simulink model "GreenCraneSimulator_SomplifiedHydMechModel"  (R2021b)
settings: Solver=ode23  StartTime=0.0  StopTime=25  FixedStep=0.0001  RelTol=1e-3
undefined symbols (not defined in the file): DiscIntNeverNeededParam, tCycle, X, Y, Z
libraries: sm_lib x25, nesl_utility x4, simulink x1
(part 1 of 2)
settings Model: Creator=hagen  LastModifiedBy=danielh

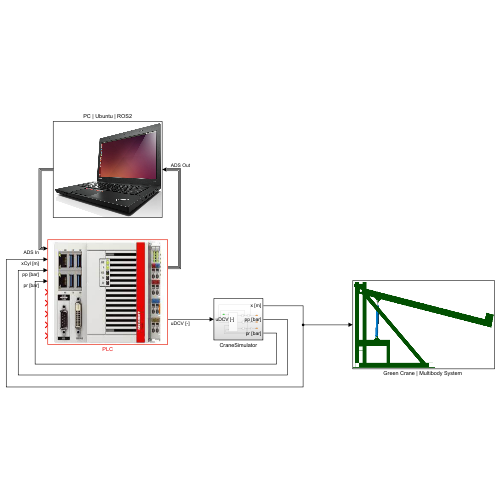
[thumbnail: Simulink's stored preview of the top-level diagram]
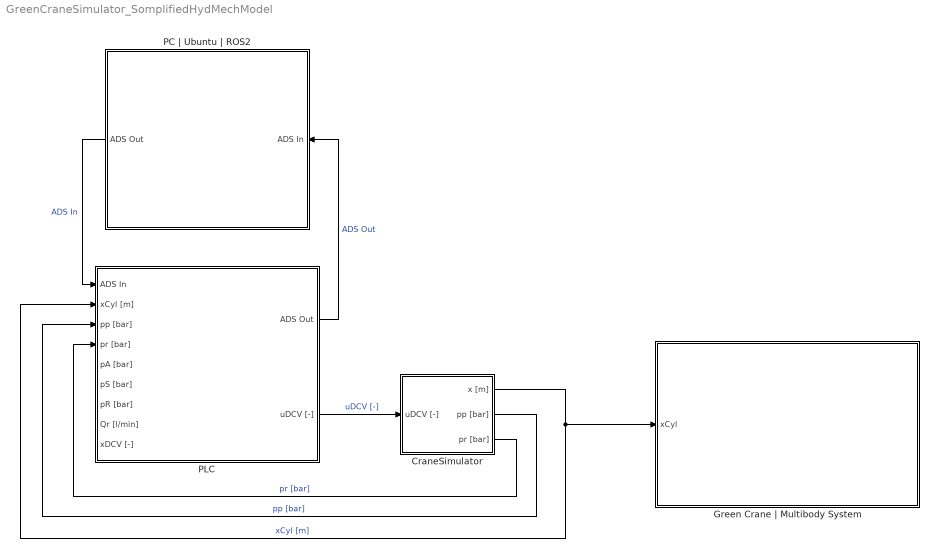
== system GreenCraneSimulator_SomplifiedHydMechModel ==
  CraneSimulator : Subsystem
  "Green Crane | Multibody System " : Subsystem
      mask Display: image('..\MAS418_SimulinkModel\Figures\GreenCrane.png'); % Use "Edit Image" on toolstrip to change.
  PC | Ubuntu | ROS2 : Subsystem
      mask Display: image('..\MAS418_SimulinkModel\Figures\PC.png'); % Use "Edit Image" on toolstrip to change.
  PLC : Subsystem
      mask Display: image('..\MAS418_SimulinkModel\Figures\PLC.jpg'); % Use "Edit Image" on toolstrip to change.
  wires:
  PC | Ubuntu | ROS2/1(ADS Out) -> PLC/1(ADS In)  "ADS In"
  CraneSimulator/2(pp [bar]) -> PLC/3(pp [bar])  "pp [bar]"
  CraneSimulator/3(pr [bar]) -> PLC/4(pr [bar])  "pr [bar]"
  PLC/1(ADS Out) -> PC | Ubuntu | ROS2/1(ADS In)  "ADS Out"
  PLC/2(uDCV [-]) -> CraneSimulator/1(uDCV [-])  "uDCV [-]"
  CraneSimulator/1(x [m]) -> PLC/2(xCyl [m]), "Green Crane | Multibody System "/1(xCyl)  "xCyl [m]"

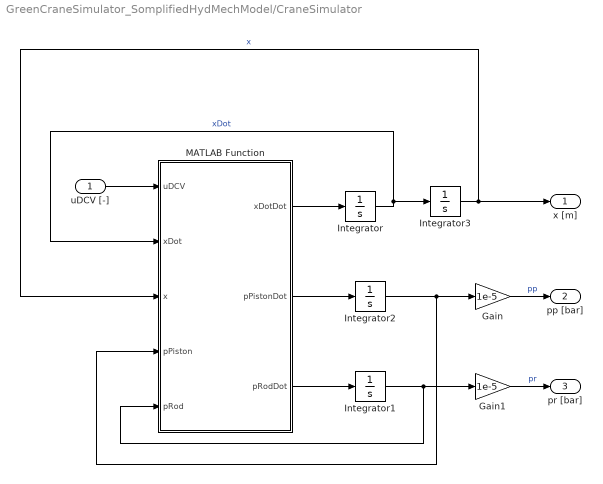
== system GreenCraneSimulator_SomplifiedHydMechModel/CraneSimulator ==
  uDCV [-] : Inport
  Gain : Gain  Gain=1e-5
  Gain1 : Gain  Gain=1e-5
  Integrator : Integrator  LimitOutput=on  UpperSaturationLimit=0.12  LowerSaturationLimit=-0.12
  Integrator1 : Integrator  InitialCondition=4.683e5  LimitOutput=on  UpperSaturationLimit=180e5  LowerSaturationLimit=1.1e5
  Integrator2 : Integrator  InitialCondition=43.77e5  LimitOutput=on  UpperSaturationLimit=180e5  LowerSaturationLimit=1.1e5
  Integrator3 : Integrator  LimitOutput=on  UpperSaturationLimit=0.5  LowerSaturationLimit=0
  MATLAB Function : MATLAB Function  TreatAsAtomicUnit=on
  x [m] : Outport
  pp [bar] : Outport  Port=2
  pr [bar] : Outport  Port=3
  wires:
  uDCV [-]/1 -> MATLAB Function/1(uDCV)
  MATLAB Function/2(pPistonDot) -> Integrator2/1
  Integrator3/1 -> x [m]/1, MATLAB Function/3(x)  "x"
  Integrator2/1 -> Gain/1, MATLAB Function/4(pPiston)
  Integrator/1 -> Integrator3/1, MATLAB Function/2(xDot)  "xDot"
  Integrator1/1 -> Gain1/1, MATLAB Function/5(pRod)
  Gain/1 -> pp [bar]/1  "pp"
  MATLAB Function/3(pRodDot) -> Integrator1/1
  MATLAB Function/1(xDotDot) -> Integrator/1
  Gain1/1 -> pr [bar]/1  "pr"

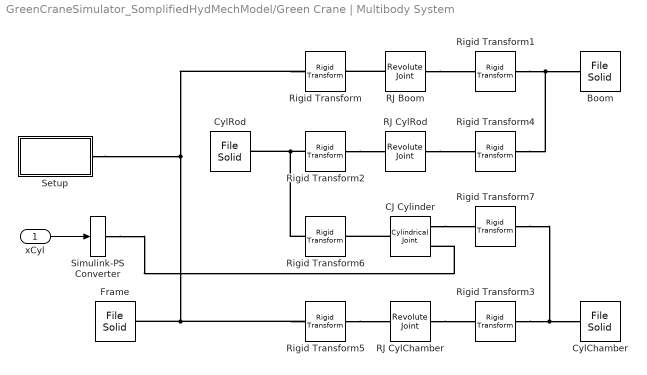
== system GreenCraneSimulator_SomplifiedHydMechModel/Green Crane | Multibody System  ==
  xCyl : Inport
  Boom : sm_lib/Body Elements/File Solid  ExtGeomFileName=..\MAS418_SimulinkModel\CAD\Boom.STL  UnitType=Custom  ExtGeomFileUnits=mm  StepReaderType=HEX  ExportConvexHullGeometry=off  InertiaType=CalculateFromGeometry  Mass=1  MassUnits=kg  CenterOfMass=[0 0 0]  CenterOfMassUnits=m  MomentsOfInertia=[1 1 1]  MomentsOfInertiaUnits=kg*m^2  ProductsOfInertia=[0 0 0]  ProductsOfInertiaUnits=kg*m^2  BasedOnType=Density  Density=1000  DensityUnits=kg/m^3  DoExposeReferenceFrame=off  SerializedFrames=<Frames><Frame><Id>Frame1</Id><Value><Name>F1</Name><Origin><Source>CenterOfMassFrame</Source><FeatureName></FeatureName></Origin><PrimaryAxis><DefinedDirection>+Y</DefinedDirection><Source>ReferenceFrame</Source><SourceDirection>-Z</SourceDirection><FeatureName></FeatureName></PrimaryAxis><SecondaryAxis><DefinedDirection>+X</DefinedDirection><Source>ReferenceFrame</Source><SourceDirection>+X</SourceDirection><FeatureName></FeatureName></SecondaryAxis></Value></Frame></Frames>  GraphicType=FromGeometry  MarkerShape=Sphere  MarkerSize=10  GraphicVisPropType=SimpleVisualProperties  GraphicDiffuseColor=[0.0 0.4 0.0]  GraphicSpecularColor=[0.5 0.5 0.5 1.0]  GraphicAmbientColor=[0.15 0.15 0.15 1.0]  GraphicEmissiveColor=[0.0 0.0 0.0 1.0]  GraphicShininess=75  GraphicOpacity=1.0
  CJ Cylinder : sm_lib/Joints/Cylindrical Joint  JointMode=Normal  SenseConstraintForce=off  SenseConstraintForceX=off  SenseConstraintForceY=off  SenseConstraintForceZ=off  SenseConstraintTorque=off  SenseConstraintTorqueX=off  SenseConstraintTorqueY=off  SenseConstraintTorqueZ=off  SenseTotalForce=off  SenseTotalForceX=off  SenseTotalForceY=off  SenseTotalForceZ=off  SenseTotalTorque=off  SenseTotalTorqueX=off  SenseTotalTorqueY=off  SenseTotalTorqueZ=off  CompositeWrenchDir=FollowerOnBase  CompositeWrenchFrame=BaseFrame  PzEquilibriumPosition=0  PzEquilibriumPositionUnits=m  PzSpringStiffness=0  PzSpringStiffnessUnits=N/m  PzDampingCoefficient=0  PzDampingCoefficientUnits=N/(m/s)  PzTorqueActuationMode=ComputedTorque  PzMotionActuationMode=InputMotion  PzSensePosition=off  PzSenseVelocity=off  PzSenseAcceleration=off  PzSenseTorqueForce=off  PzSenseLowerLimitTorqueForce=off  PzSenseUpperLimitTorqueForce=off  PzLowerLimitSpecify=off  PzLowerLimitBound=-1  PzLowerLimitBoundUnits=m  PzLowerLimitStiffness=1e6  PzLowerLimitStiffnessUnits=N/m  PzLowerLimitDamping=1e3  PzLowerLimitDampingUnits=N/(m/s)  PzLowerLimitTransitionRegionWidth=1e-4  PzLowerLimitTransitionRegionWidthUnits=m  PzUpperLimitSpecify=off  PzUpperLimitBound=1  PzUpperLimitBoundUnits=m  PzUpperLimitStiffness=1e6  PzUpperLimitStiffnessUnits=N/m  PzUpperLimitDamping=1e3  PzUpperLimitDampingUnits=N/(m/s)  PzUpperLimitTransitionRegionWidth=1e-4  PzUpperLimitTransitionRegionWidthUnits=m  PzPositionTargetSpecify=on  PzPositionTargetPriority=High  PzPositionTargetValue=0  PzPositionTargetValueUnits=m  PzVelocityTargetSpecify=off  PzVelocityTargetPriority=High  PzVelocityTargetValue=0  PzVelocityTargetValueUnits=m/s  RzEquilibriumPosition=0  RzEquilibriumPositionUnits=deg  RzSpringStiffness=0  RzSpringStiffnessUnits=N*m/deg  RzDampingCoefficient=0  RzDampingCoefficientUnits=N*m/(deg/s)  RzTorqueActuationMode=NoTorque  RzMotionActuationMode=ComputedMotion  RzSensePosition=off  RzSenseVelocity=off  RzSenseAcceleration=off  RzSenseTorqueForce=off  RzSenseLowerLimitTorqueForce=off  RzSenseUpperLimitTorqueForce=off  RzLowerLimitSpecify=off  RzLowerLimitBound=-90  RzLowerLimitBoundUnits=deg  RzLowerLimitStiffness=1e4  RzLowerLimitStiffnessUnits=N*m/deg  RzLowerLimitDamping=10  RzLowerLimitDampingUnits=N*m/(deg/s)  RzLowerLimitTransitionRegionWidth=0.1  RzLowerLimitTransitionRegionWidthUnits=deg  RzUpperLimitSpecify=off  RzUpperLimitBound=90  RzUpperLimitBoundUnits=deg  RzUpperLimitStiffness=1e4  RzUpperLimitStiffnessUnits=N*m/deg  RzUpperLimitDamping=10  RzUpperLimitDampingUnits=N*m/(deg/s)  RzUpperLimitTransitionRegionWidth=0.1  RzUpperLimitTransitionRegionWidthUnits=deg  RzPositionTargetSpecify=off  RzPositionTargetPriority=High  RzPositionTargetValue=0  RzPositionTargetValueUnits=deg  RzVelocityTargetSpecify=off  RzVelocityTargetPriority=High  RzVelocityTargetValue=0  RzVelocityTargetValueUnits=deg/s
  CylChamber : sm_lib/Body Elements/File Solid  ExtGeomFileName=..\MAS418_SimulinkModel\CAD\cyl_chamber.STL  UnitType=Custom  ExtGeomFileUnits=mm  StepReaderType=HEX  ExportConvexHullGeometry=off  InertiaType=CalculateFromGeometry  Mass=1  MassUnits=kg  CenterOfMass=[0 0 0]  CenterOfMassUnits=m  MomentsOfInertia=[1 1 1]  MomentsOfInertiaUnits=kg*m^2  ProductsOfInertia=[0 0 0]  ProductsOfInertiaUnits=kg*m^2  BasedOnType=Density  Density=1000  DensityUnits=kg/m^3  DoExposeReferenceFrame=off  SerializedFrames=<Frames><Frame><Id>Frame1</Id><Value><Name>F1</Name><Origin><Source>CenterOfMassFrame</Source><FeatureName></FeatureName></Origin><PrimaryAxis><DefinedDirection>+Y</DefinedDirection><Source>ReferenceFrame</Source><SourceDirection>-Z</SourceDirection><FeatureName></FeatureName></PrimaryAxis><SecondaryAxis><DefinedDirection>+X</DefinedDirection><Source>ReferenceFrame</Source><SourceDirection>+X</SourceDirection><FeatureName></FeatureName></SecondaryAxis></Value></Frame></Frames>  GraphicType=FromGeometry  MarkerShape=Sphere  MarkerSize=10  GraphicVisPropType=SimpleVisualProperties  GraphicDiffuseColor=[0.0 0.6 1.0]  GraphicSpecularColor=[0.5 0.5 0.5 1.0]  GraphicAmbientColor=[0.15 0.15 0.15 1.0]  GraphicEmissiveColor=[0.0 0.0 0.0 1.0]  GraphicShininess=75  GraphicOpacity=1.0
  CylRod : sm_lib/Body Elements/File Solid  ExtGeomFileName=..\MAS418_SimulinkModel\CAD\cyl_rod.STL  UnitType=Custom  ExtGeomFileUnits=mm  StepReaderType=HEX  ExportConvexHullGeometry=off  InertiaType=CalculateFromGeometry  Mass=1  MassUnits=kg  CenterOfMass=[0 0 0]  CenterOfMassUnits=m  MomentsOfInertia=[1 1 1]  MomentsOfInertiaUnits=kg*m^2  ProductsOfInertia=[0 0 0]  ProductsOfInertiaUnits=kg*m^2  BasedOnType=Density  Density=1000  DensityUnits=kg/m^3  DoExposeReferenceFrame=off  SerializedFrames=<Frames><Frame><Id>Frame1</Id><Value><Name>F1</Name><Origin><Source>CenterOfMassFrame</Source><FeatureName></FeatureName></Origin><PrimaryAxis><DefinedDirection>+Y</DefinedDirection><Source>ReferenceFrame</Source><SourceDirection>-Z</SourceDirection><FeatureName></FeatureName></PrimaryAxis><SecondaryAxis><DefinedDirection>+X</DefinedDirection><Source>ReferenceFrame</Source><SourceDirection>+X</SourceDirection><FeatureName></FeatureName></SecondaryAxis></Value></Frame></Frames>  GraphicType=FromGeometry  MarkerShape=Sphere  MarkerSize=10  GraphicVisPropType=SimpleVisualProperties  GraphicDiffuseColor=[0.8 0.8 0.8]  GraphicSpecularColor=[0.5 0.5 0.5 1.0]  GraphicAmbientColor=[0.15 0.15 0.15 1.0]  GraphicEmissiveColor=[0.0 0.0 0.0 1.0]  GraphicShininess=75  GraphicOpacity=1.0
  Frame : sm_lib/Body Elements/File Solid  ExtGeomFileName=..\MAS418_SimulinkModel\CAD\Frame.STL  UnitType=Custom  ExtGeomFileUnits=mm  StepReaderType=HEX  ExportConvexHullGeometry=off  InertiaType=CalculateFromGeometry  Mass=1  MassUnits=kg  CenterOfMass=[0 0 0]  CenterOfMassUnits=m  MomentsOfInertia=[1 1 1]  MomentsOfInertiaUnits=kg*m^2  ProductsOfInertia=[0 0 0]  ProductsOfInertiaUnits=kg*m^2  BasedOnType=Density  Density=1000  DensityUnits=kg/m^3  DoExposeReferenceFrame=off  SerializedFrames=<Frames><Frame><Id>Frame1</Id><Value><Name>F1</Name><Origin><Source>CenterOfMassFrame</Source><FeatureName></FeatureName></Origin><PrimaryAxis><DefinedDirection>-Y</DefinedDirection><Source>ReferenceFrame</Source><SourceDirection>+Z</SourceDirection><FeatureName></FeatureName></PrimaryAxis><SecondaryAxis><DefinedDirection>+X</DefinedDirection><Source>ReferenceFrame</Source><SourceDirection>+X</SourceDirection><FeatureName></FeatureName></SecondaryAxis></Value></Frame></Frames>  GraphicType=FromGeometry  MarkerShape=Sphere  MarkerSize=10  GraphicVisPropType=SimpleVisualProperties  GraphicDiffuseColor=[0.0 0.4 0.0]  GraphicSpecularColor=[0.5 0.5 0.5 1.0]  GraphicAmbientColor=[0.15 0.15 0.15 1.0]  GraphicEmissiveColor=[0.0 0.0 0.0 1.0]  GraphicShininess=75  GraphicOpacity=1.0
  RJ Boom : sm_lib/Joints/Revolute Joint  JointMode=Normal  SenseConstraintForce=off  SenseConstraintForceX=off  SenseConstraintForceY=off  SenseConstraintForceZ=off  SenseConstraintTorque=off  SenseConstraintTorqueX=off  SenseConstraintTorqueY=off  SenseConstraintTorqueZ=off  SenseTotalForce=off  SenseTotalForceX=off  SenseTotalForceY=off  SenseTotalForceZ=off  SenseTotalTorque=off  SenseTotalTorqueX=off  SenseTotalTorqueY=off  SenseTotalTorqueZ=off  CompositeWrenchDir=FollowerOnBase  CompositeWrenchFrame=BaseFrame  EquilibriumPosition=0  EquilibriumPositionUnits=deg  SpringStiffness=0  SpringStiffnessUnits=N*m/deg  DampingCoefficient=0  DampingCoefficientUnits=N*m/(deg/s)  TorqueActuationMode=NoTorque  MotionActuationMode=ComputedMotion  SensePosition=off  SenseVelocity=off  SenseAcceleration=off  SenseTorqueForce=off  SenseLowerLimitTorqueForce=off  SenseUpperLimitTorqueForce=off  LowerLimitSpecify=off  LowerLimitBound=-90  LowerLimitBoundUnits=deg  LowerLimitStiffness=1e4  LowerLimitStiffnessUnits=N*m/deg  LowerLimitDamping=10  LowerLimitDampingUnits=N*m/(deg/s)  LowerLimitTransitionRegionWidth=0.1  LowerLimitTransitionRegionWidthUnits=deg  UpperLimitSpecify=off  UpperLimitBound=90  UpperLimitBoundUnits=deg  UpperLimitStiffness=1e4  UpperLimitStiffnessUnits=N*m/deg  UpperLimitDamping=10  UpperLimitDampingUnits=N*m/(deg/s)  UpperLimitTransitionRegionWidth=0.1  UpperLimitTransitionRegionWidthUnits=deg  PositionTargetSpecify=off  PositionTargetPriority=High  PositionTargetValue=0  PositionTargetValueUnits=deg  VelocityTargetSpecify=off  VelocityTargetPriority=High  VelocityTargetValue=0  VelocityTargetValueUnits=deg/s
  RJ CylChamber : sm_lib/Joints/Revolute Joint  JointMode=Normal  SenseConstraintForce=off  SenseConstraintForceX=off  SenseConstraintForceY=off  SenseConstraintForceZ=off  SenseConstraintTorque=off  SenseConstraintTorqueX=off  SenseConstraintTorqueY=off  SenseConstraintTorqueZ=off  SenseTotalForce=off  SenseTotalForceX=off  SenseTotalForceY=off  SenseTotalForceZ=off  SenseTotalTorque=off  SenseTotalTorqueX=off  SenseTotalTorqueY=off  SenseTotalTorqueZ=off  CompositeWrenchDir=FollowerOnBase  CompositeWrenchFrame=BaseFrame  EquilibriumPosition=0  EquilibriumPositionUnits=deg  SpringStiffness=0  SpringStiffnessUnits=N*m/deg  DampingCoefficient=0  DampingCoefficientUnits=N*m/(deg/s)  TorqueActuationMode=NoTorque  MotionActuationMode=ComputedMotion  SensePosition=off  SenseVelocity=off  SenseAcceleration=off  SenseTorqueForce=off  SenseLowerLimitTorqueForce=off  SenseUpperLimitTorqueForce=off  LowerLimitSpecify=off  LowerLimitBound=-90  LowerLimitBoundUnits=deg  LowerLimitStiffness=1e4  LowerLimitStiffnessUnits=N*m/deg  LowerLimitDamping=10  LowerLimitDampingUnits=N*m/(deg/s)  LowerLimitTransitionRegionWidth=0.1  LowerLimitTransitionRegionWidthUnits=deg  UpperLimitSpecify=off  UpperLimitBound=90  UpperLimitBoundUnits=deg  UpperLimitStiffness=1e4  UpperLimitStiffnessUnits=N*m/deg  UpperLimitDamping=10  UpperLimitDampingUnits=N*m/(deg/s)  UpperLimitTransitionRegionWidth=0.1  UpperLimitTransitionRegionWidthUnits=deg  PositionTargetSpecify=off  PositionTargetPriority=High  PositionTargetValue=0  PositionTargetValueUnits=deg  VelocityTargetSpecify=off  VelocityTargetPriority=High  VelocityTargetValue=0  VelocityTargetValueUnits=deg/s
  RJ CylRod : sm_lib/Joints/Revolute Joint  JointMode=Normal  SenseConstraintForce=off  SenseConstraintForceX=off  SenseConstraintForceY=off  SenseConstraintForceZ=off  SenseConstraintTorque=off  SenseConstraintTorqueX=off  SenseConstraintTorqueY=off  SenseConstraintTorqueZ=off  SenseTotalForce=off  SenseTotalForceX=off  SenseTotalForceY=off  SenseTotalForceZ=off  SenseTotalTorque=off  SenseTotalTorqueX=off  SenseTotalTorqueY=off  SenseTotalTorqueZ=off  CompositeWrenchDir=FollowerOnBase  CompositeWrenchFrame=BaseFrame  EquilibriumPosition=0  EquilibriumPositionUnits=deg  SpringStiffness=0  SpringStiffnessUnits=N*m/deg  DampingCoefficient=0  DampingCoefficientUnits=N*m/(deg/s)  TorqueActuationMode=NoTorque  MotionActuationMode=ComputedMotion  SensePosition=off  SenseVelocity=off  SenseAcceleration=off  SenseTorqueForce=off  SenseLowerLimitTorqueForce=off  SenseUpperLimitTorqueForce=off  LowerLimitSpecify=off  LowerLimitBound=-90  LowerLimitBoundUnits=deg  LowerLimitStiffness=1e4  LowerLimitStiffnessUnits=N*m/deg  LowerLimitDamping=10  LowerLimitDampingUnits=N*m/(deg/s)  LowerLimitTransitionRegionWidth=0.1  LowerLimitTransitionRegionWidthUnits=deg  UpperLimitSpecify=off  UpperLimitBound=90  UpperLimitBoundUnits=deg  UpperLimitStiffness=1e4  UpperLimitStiffnessUnits=N*m/deg  UpperLimitDamping=10  UpperLimitDampingUnits=N*m/(deg/s)  UpperLimitTransitionRegionWidth=0.1  UpperLimitTransitionRegionWidthUnits=deg  PositionTargetSpecify=off  PositionTargetPriority=High  PositionTargetValue=0  PositionTargetValueUnits=deg  VelocityTargetSpecify=off  VelocityTargetPriority=High  VelocityTargetValue=0  VelocityTargetValueUnits=deg/s
  Rigid Transform : sm_lib/Frames and Transforms/Rigid Transform  TranslationMethod=Cartesian  TranslationStandardOffset=0  TranslationLengthUnit=mm  TranslationStandardAxis=+Z  TranslationCartesianOffset=[-568.76 0 1179.93]  TranslationROffset=0  TranslationROffsetUnits=m  TranslationZOffset=0  TranslationZOffsetUnits=m  TranslationThetaOffset=0  TranslationThetaOffsetUnits=deg  RotationMethod=StandardAxis  RotationAngleUnits=deg  RotationStandardAxis=+X  RotationAngle=90  RotationArbitraryAxis=[0 0 1]  FollAlignAxisA=+X  BaseAlignAxisA=+Y  FollAlignAxisB=+Y  BaseAlignAxisB=+Z  RotationSequenceAxes=FollowerAxes  RotationSequence=XYX  RotationSequenceAngles=[0 0 0]  RotationSequenceAnglesUnits=deg  RotationMatrix=[1 0 0; 0 1 0; 0 0 1]
  Rigid Transform1 : sm_lib/Frames and Transforms/Rigid Transform  TranslationMethod=Cartesian  TranslationStandardOffset=0  TranslationLengthUnit=mm  TranslationStandardAxis=+Z  TranslationCartesianOffset=[-3108.36 0 -63.43]  TranslationROffset=0  TranslationROffsetUnits=m  TranslationZOffset=0  TranslationZOffsetUnits=m  TranslationThetaOffset=0  TranslationThetaOffsetUnits=deg  RotationMethod=StandardAxis  RotationAngleUnits=deg  RotationStandardAxis=+X  RotationAngle=90  RotationArbitraryAxis=[0 0 1]  FollAlignAxisA=+X  BaseAlignAxisA=+Y  FollAlignAxisB=+Y  BaseAlignAxisB=+Z  RotationSequenceAxes=FollowerAxes  RotationSequence=XYX  RotationSequenceAngles=[0 0 0]  RotationSequenceAnglesUnits=deg  RotationMatrix=[1 0 0; 0 1 0; 0 0 1]
  Rigid Transform2 : sm_lib/Frames and Transforms/Rigid Transform  TranslationMethod=Cartesian  TranslationStandardOffset=0  TranslationLengthUnit=mm  TranslationStandardAxis=+Z  TranslationCartesianOffset=[0 0 292.43]  TranslationROffset=0  TranslationROffsetUnits=m  TranslationZOffset=0  TranslationZOffsetUnits=m  TranslationThetaOffset=0  TranslationThetaOffsetUnits=deg  RotationMethod=StandardAxis  RotationAngleUnits=deg  RotationStandardAxis=+X  RotationAngle=90  RotationArbitraryAxis=[0 0 1]  FollAlignAxisA=+X  BaseAlignAxisA=+Y  FollAlignAxisB=+Y  BaseAlignAxisB=+Z  RotationSequenceAxes=FollowerAxes  RotationSequence=XYX  RotationSequenceAngles=[0 0 0]  RotationSequenceAnglesUnits=deg  RotationMatrix=[1 0 0; 0 1 0; 0 0 1]
  Rigid Transform3 : sm_lib/Frames and Transforms/Rigid Transform  TranslationMethod=Cartesian  TranslationStandardOffset=0  TranslationLengthUnit=mm  TranslationStandardAxis=+Z  TranslationCartesianOffset=[0 0 -260.99]  TranslationROffset=0  TranslationROffsetUnits=m  TranslationZOffset=0  TranslationZOffsetUnits=m  TranslationThetaOffset=0  TranslationThetaOffsetUnits=deg  RotationMethod=StandardAxis  RotationAngleUnits=deg  RotationStandardAxis=+X  RotationAngle=90  RotationArbitraryAxis=[0 0 1]  FollAlignAxisA=+X  BaseAlignAxisA=+Y  FollAlignAxisB=+Y  BaseAlignAxisB=+Z  RotationSequenceAxes=FollowerAxes  RotationSequence=XYX  RotationSequenceAngles=[0 0 0]  RotationSequenceAnglesUnits=deg  RotationMatrix=[1 0 0; 0 1 0; 0 0 1]
  Rigid Transform4 : sm_lib/Frames and Transforms/Rigid Transform  TranslationMethod=Cartesian  TranslationStandardOffset=0  TranslationLengthUnit=mm  TranslationStandardAxis=+Z  TranslationCartesianOffset=[-2613.52 0 -196.43]  TranslationROffset=0  TranslationROffsetUnits=m  TranslationZOffset=0  TranslationZOffsetUnits=m  TranslationThetaOffset=0  TranslationThetaOffsetUnits=deg  RotationMethod=StandardAxis  RotationAngleUnits=deg  RotationStandardAxis=+X  RotationAngle=90  RotationArbitraryAxis=[0 0 1]  FollAlignAxisA=+X  BaseAlignAxisA=+Y  FollAlignAxisB=+Y  BaseAlignAxisB=+Z  RotationSequenceAxes=FollowerAxes  RotationSequence=XYX  RotationSequenceAngles=[0 0 0]  RotationSequenceAnglesUnits=deg  RotationMatrix=[1 0 0; 0 1 0; 0 0 1]
  Rigid Transform5 : sm_lib/Frames and Transforms/Rigid Transform  TranslationMethod=Cartesian  TranslationStandardOffset=0  TranslationLengthUnit=mm  TranslationStandardAxis=+Z  TranslationCartesianOffset=[-141.76 0 122.93]  TranslationROffset=0  TranslationROffsetUnits=m  TranslationZOffset=0  TranslationZOffsetUnits=m  TranslationThetaOffset=0  TranslationThetaOffsetUnits=deg  RotationMethod=StandardAxis  RotationAngleUnits=deg  RotationStandardAxis=+X  RotationAngle=90  RotationArbitraryAxis=[0 0 1]  FollAlignAxisA=+X  BaseAlignAxisA=+Y  FollAlignAxisB=+Y  BaseAlignAxisB=+Z  RotationSequenceAxes=FollowerAxes  RotationSequence=XYX  RotationSequenceAngles=[0 0 0]  RotationSequenceAnglesUnits=deg  RotationMatrix=[1 0 0; 0 1 0; 0 0 1]
  Rigid Transform6 : sm_lib/Frames and Transforms/Rigid Transform  TranslationMethod=Cartesian  TranslationStandardOffset=0  TranslationLengthUnit=mm  TranslationStandardAxis=+Z  TranslationCartesianOffset=[0 0 -307.79]  TranslationROffset=0  TranslationROffsetUnits=m  TranslationZOffset=0  TranslationZOffsetUnits=m  TranslationThetaOffset=0  TranslationThetaOffsetUnits=deg  RotationMethod=None  RotationAngleUnits=deg  RotationStandardAxis=-X  RotationAngle=90  RotationArbitraryAxis=[0 0 1]  FollAlignAxisA=+X  BaseAlignAxisA=+Y  FollAlignAxisB=+Y  BaseAlignAxisB=+Z  RotationSequenceAxes=FollowerAxes  RotationSequence=XYX  RotationSequenceAngles=[0 0 0]  RotationSequenceAnglesUnits=deg  RotationMatrix=[1 0 0; 0 1 0; 0 0 1]
  Rigid Transform7 : sm_lib/Frames and Transforms/Rigid Transform  TranslationMethod=Cartesian  TranslationStandardOffset=0  TranslationLengthUnit=mm  TranslationStandardAxis=+Z  TranslationCartesianOffset=[0 0 -88.99]  TranslationROffset=0  TranslationROffsetUnits=m  TranslationZOffset=0  TranslationZOffsetUnits=m  TranslationThetaOffset=0  TranslationThetaOffsetUnits=deg  RotationMethod=None  RotationAngleUnits=deg  RotationStandardAxis=-X  RotationAngle=90  RotationArbitraryAxis=[0 0 1]  FollAlignAxisA=+X  BaseAlignAxisA=+Y  FollAlignAxisB=+Y  BaseAlignAxisB=+Z  RotationSequenceAxes=FollowerAxes  RotationSequence=XYX  RotationSequenceAngles=[0 0 0]  RotationSequenceAnglesUnits=deg  RotationMatrix=[1 0 0; 0 1 0; 0 0 1]
  Setup : Subsystem
  Simulink-PS Converter : nesl_utility/Simulink-PS Converter  PhysicalDomain=network_engine_domain  SubClassName=ps_input  LeftPortType=input  RightPortType=output  PseudoPeriodic=off  Frequencies=[]  NoiseDistribution=none  NoiseParameters=[]  Unit=1  AffineConversion=off  FilteringAndDerivatives=filter  SimscapeFilterOrder=2  InputFilterTimeConstant=0.001  UdotUserProvided=0
      settings: SourceProductBaseCode=PW,SS
  wires:
  xCyl/1 -> Simulink-PS Converter/1
  connections:
  Rigid Transform/LConn1 -- Rigid Transform5/LConn1 -- Frame/LConn1 -- Setup/RConn1
  CJ Cylinder/LConn1 -- Rigid Transform7/RConn1
  Rigid Transform2/LConn1 -- Rigid Transform6/LConn1 -- CylRod/LConn1
  Rigid Transform1/LConn1 -- Rigid Transform4/LConn1 -- Boom/LConn1
  Rigid Transform3/LConn1 -- Rigid Transform7/LConn1 -- CylChamber/LConn1
  RJ CylChamber/RConn1 -- Rigid Transform3/RConn1
  RJ Boom/LConn1 -- Rigid Transform/RConn1
  CJ Cylinder/RConn1 -- Rigid Transform6/RConn1
  RJ Boom/RConn1 -- Rigid Transform1/RConn1
  Simulink-PS Converter/RConn1 -- CJ Cylinder/LConn2
  Rigid Transform5/RConn1 -- RJ CylChamber/LConn1
  RJ CylRod/LConn1 -- Rigid Transform4/RConn1
  Rigid Transform2/RConn1 -- RJ CylRod/RConn1

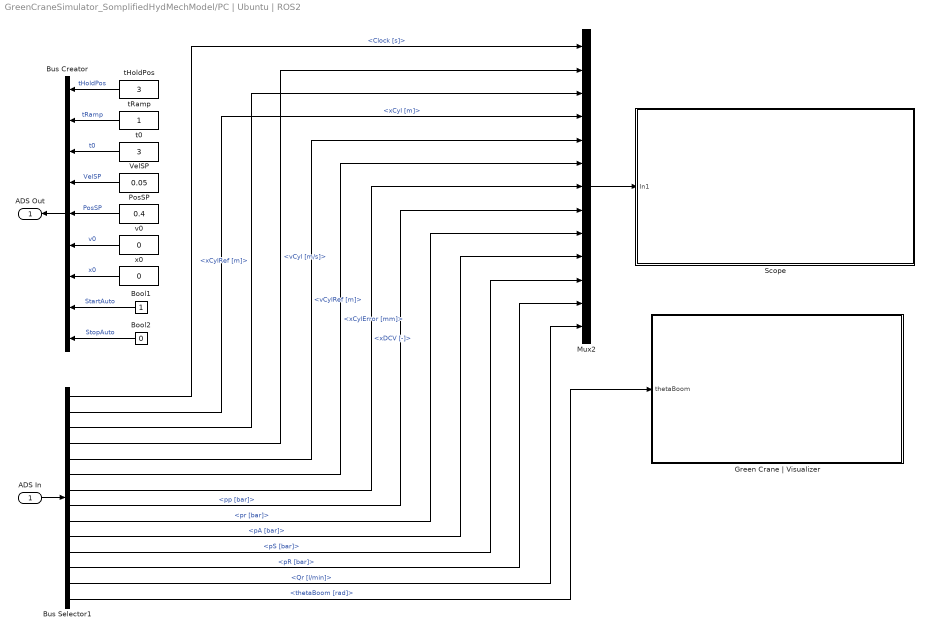
== system GreenCraneSimulator_SomplifiedHydMechModel/PC | Ubuntu | ROS2 ==
  ADS In : Inport
  Bool1 : Constant  OutDataTypeStr=boolean
  Bool2 : Constant  Value=0  OutDataTypeStr=boolean
  Bus Creator : BusCreator  Inputs=9
  Bus Selector1 : BusSelector  OutputSignals=Clock [s],xCyl [m],xCylRef [m],vCyl [m/s],vCylRef [m],xCylError [mm],xDCV [-],pp [bar],pr [bar],pA [bar],pS [bar],pR [bar],Qr [l/min],thetaBoom [rad]
  "Green Crane | Visualizer " : Subsystem
      mask Display: image('..\MAS418_SimulinkModel\Figures\GreenCraneSimple.png'); % Use "Edit Image" on toolstrip to change.
  Mux2 : Mux  Inputs=13
  PosSP : Constant  Value=0.4  OutDataTypeStr=double
  Scope : Subsystem
      mask Display: image('..\MAS418_SimulinkModel\Figures\Scope.png'); % Use "Edit Image" on toolstrip to change.
  VelSP : Constant  Value=0.05  OutDataTypeStr=double
  t0 : Constant  Value=3  OutDataTypeStr=double
  tHoldPos : Constant  Value=3  OutDataTypeStr=double
  tRamp : Constant  OutDataTypeStr=double
  v0 : Constant  Value=0  OutDataTypeStr=double
  x0 : Constant  Value=0  OutDataTypeStr=double
  ADS Out : Outport
  wires:
  Bus Selector1/1 -> Mux2/1  "<Clock [s]>"
  Bus Selector1/2 -> Mux2/4  "<xCyl [m]>"
  Bus Selector1/4 -> Mux2/2  "<vCyl [m/s]>"
  Bus Creator/1 -> ADS Out/1
  ADS In/1 -> Bus Selector1/1
  Bus Selector1/8 -> Mux2/8  "<pp [bar]>"
  Bus Selector1/9 -> Mux2/9  "<pr [bar]>"
  Bus Selector1/6 -> Mux2/6  "<xCylError [mm]>"
  Mux2/1 -> Scope/1(In1)
  Bus Selector1/10 -> Mux2/10  "<pA [bar]>"
  Bus Selector1/11 -> Mux2/11  "<pS [bar]>"
  Bus Selector1/12 -> Mux2/12  "<pR [bar]>"
  Bus Selector1/13 -> Mux2/13  "<Qr [l/min]>"
  Bus Selector1/7 -> Mux2/7  "<xDCV [-]>"
  Bus Selector1/14 -> "Green Crane | Visualizer "/1(thetaBoom)  "<thetaBoom [rad]>"
  tHoldPos/1 -> Bus Creator/1  "tHoldPos"
  tRamp/1 -> Bus Creator/2  "tRamp"
  t0/1 -> Bus Creator/3  "t0"
  VelSP/1 -> Bus Creator/4  "VelSP"
  PosSP/1 -> Bus Creator/5  "PosSP"
  v0/1 -> Bus Creator/6  "v0"
  x0/1 -> Bus Creator/7  "x0"
  Bus Selector1/3 -> Mux2/3  "<xCylRef [m]>"
  Bus Selector1/5 -> Mux2/5  "<vCylRef [m]>"
  Bool1/1 -> Bus Creator/8  "StartAuto"
  Bool2/1 -> Bus Creator/9  "StopAuto"

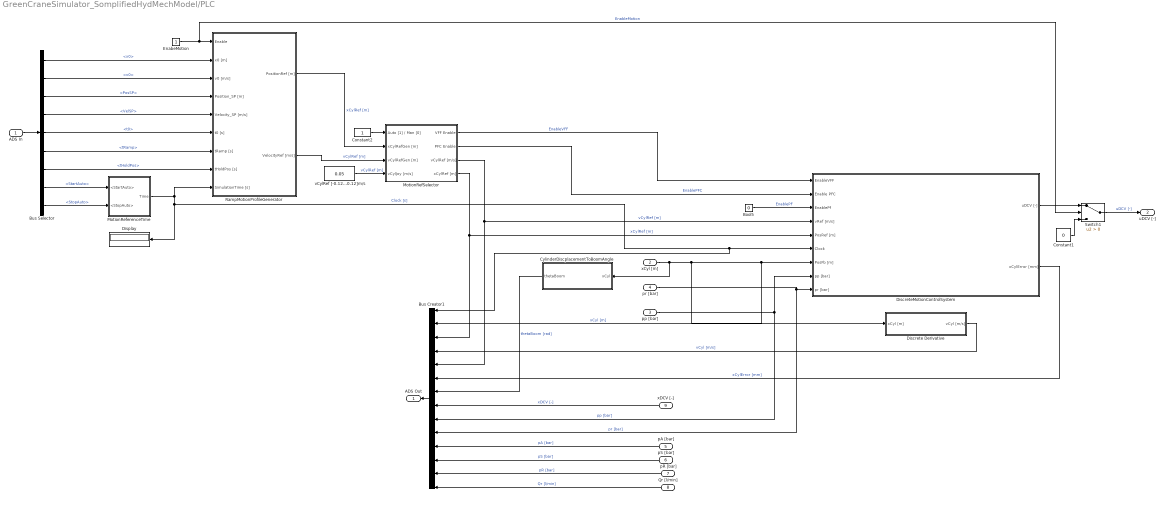
== system GreenCraneSimulator_SomplifiedHydMechModel/PLC ==
  ADS In : Inport
  xCyl [m] : Inport  Port=2
  pp [bar] : Inport  Port=3
  pr [bar] : Inport  Port=4
  pA [bar] : Inport  Port=5
  pS [bar] : Inport  Port=6
  pR [bar] : Inport  Port=7
  Qr [l/min] : Inport  Port=8
  xDCV [-] : Inport  Port=9
  Bool5 : Constant  Value=0  OutDataTypeStr=boolean
  Bus Creator1 : BusCreator  Inputs=14
  Bus Selector : BusSelector  OutputSignals=x0,v0,PosSP,VelSP,t0,tRamp,tHoldPos,StartAuto,StopAuto
  Constant1 : Constant  Value=0
  Constant2 : Constant  OutDataTypeStr=boolean
  CylinderDiscplacementToBoomAngle : MATLAB Function  TreatAsAtomicUnit=on
  Discrete Derivative : Subsystem
  DiscreteMotionControlSystem : Subsystem
      mask Display: image('..\MAS418_SimulinkModel\Figures\MotionControlSystem.png'); % Use "Edit Image" on toolstrip to change.
  Display : Display
  EnabeMotion : Constant  OutDataTypeStr=boolean
  MotionRefSelector : Subsystem
  MotionReferenceTime : Subsystem
  RampMotionProfileGenerator : Subsystem  TreatAsAtomicUnit=on  VariantControl=Ramp_Profile
  Switch1 : Switch  Criteria=u2 > Threshold
  vCylRef [-0.12...0.12]m/s : Constant  Value=0.05  OutDataTypeStr=double
  ADS Out : Outport
  uDCV [-] : Outport  Port=2
  wires:
  Switch1/1 -> uDCV [-]/1  "uDCV [-]"
  xCyl [m]/1 -> CylinderDiscplacementToBoomAngle/1(xCyl), Discrete Derivative/1(xCyl [m]), Bus Creator1/2, DiscreteMotionControlSystem/7(PosFb [m])  "xCyl [m]"
  pr [bar]/1 -> Bus Creator1/10, DiscreteMotionControlSystem/9(pr [bar])  "pr [bar]"
  MotionReferenceTime/1(Time) -> Bus Creator1/1, DiscreteMotionControlSystem/6(Clock), Display/1, RampMotionProfileGenerator/9(SimulationTime [s])  "Clock [s]"
  pp [bar]/1 -> Bus Creator1/9, DiscreteMotionControlSystem/8(pp [bar])  "pp [bar]"
  Bus Creator1/1 -> ADS Out/1
  ADS In/1 -> Bus Selector/1
  Constant1/1 -> Switch1/3
  DiscreteMotionControlSystem/1(uDCV [-]) -> Switch1/1
  DiscreteMotionControlSystem/2(xCylError [mm]) -> Bus Creator1/6  "xCylError [mm]"
  Discrete Derivative/1(vCyl [m/s]) -> Bus Creator1/4  "vCyl [m/s]"
  xDCV [-]/1 -> Bus Creator1/8  "xDCV [-]"
  pA [bar]/1 -> Bus Creator1/11  "pA [bar]"
  pS [bar]/1 -> Bus Creator1/12  "pS [bar]"
  pR [bar]/1 -> Bus Creator1/13  "pR [bar]"
  Qr [l/min]/1 -> Bus Creator1/14  "Qr [l/min]"
  CylinderDiscplacementToBoomAngle/1(thetaBoom) -> Bus Creator1/7  "thetaBoom [rad]"
  vCylRef [-0.12...0.12]m/s/1 -> MotionRefSelector/4(vCylJoy [m/s])  "vCylRef [m]"
  Bus Selector/1 -> RampMotionProfileGenerator/2(x0 [m])  "<x0>"
  Constant2/1 -> MotionRefSelector/1(Auto [1] / Man [0])
  RampMotionProfileGenerator/1("PositionRef [m] ") -> MotionRefSelector/2(xCylRefGen [m])  "xCylRef [m]"
  Bus Selector/5 -> RampMotionProfileGenerator/6(t0 [s])  "<t0>"
  MotionRefSelector/3(vCylRef [m/s]) -> Bus Creator1/5, DiscreteMotionControlSystem/4(vRef [m/s])  "vCylRef [m]"
  Bus Selector/2 -> RampMotionProfileGenerator/3(v0 [m/s])  "<v0>"
  RampMotionProfileGenerator/2(VelocityRef [m/s]) -> MotionRefSelector/3(vCylRefGen [m])  "vCylRef [m]"
  Bus Selector/7 -> RampMotionProfileGenerator/8(tHoldPos [s])  "<tHoldPos>"
  Bus Selector/3 -> RampMotionProfileGenerator/4(Position_SP [m])  "<PosSP>"
  Bus Selector/4 -> RampMotionProfileGenerator/5("Velocity_SP [m/s] ")  "<VelSP>"
  MotionRefSelector/4(xCylRef [m]) -> Bus Creator1/3, DiscreteMotionControlSystem/5(PosRef [m])  "xCylRef [m]"
  Bus Selector/6 -> RampMotionProfileGenerator/7(tRamp [s])  "<tRamp>"
  MotionRefSelector/1(VFF Enable) -> DiscreteMotionControlSystem/1(EnableVFF)  "EnableVFF"
  MotionRefSelector/2(PFC Enable) -> DiscreteMotionControlSystem/2(Enable PFC)  "EnablePFC"
  Bool5/1 -> DiscreteMotionControlSystem/3(EnablePf)  "EnablePF"
  EnabeMotion/1 -> RampMotionProfileGenerator/1(Enable), Switch1/2  "EnableMotion"
  Bus Selector/8 -> MotionReferenceTime/1(<StartAuto>)  "<StartAuto>"
  Bus Selector/9 -> MotionReferenceTime/2(<StopAuto>)  "<StopAuto>"

== system GreenCraneSimulator_SomplifiedHydMechModel/Green Crane | Multibody System /Setup ==
  Mechanism Configuration1 : sm_lib/Utilities/Mechanism Configuration  UniformGravity=Constant  GravityVector=[0 0 -9.80665]  GravityUnits=m/s^2  LinearizationDelta=0.001  JointModeTransitionNonlinearIterations=2
  Solver Configuration : nesl_utility/Solver Configuration  PhysicalDomain=network_engine_domain  SubClassName=solver  LeftPortType=input  RightPortType=generic  Tones=[]  Harmonics=[]  SimulateNoise=off  Profile=off  UseLocalSampling=off  EnableSwitchedLinearOptims=on  FrequencyDomain=off  UseCCode=off  RelTol=0.001  AbsTol=1e-06  MinStep=1e-09  ToWorkspace=off  RevertToSquareIcSolve=off  NumHomotopyIterations=100  PhasorMode=off  PhasorModeNumHarmonics=1  DoDC=off  ResidualTolerance=1e-09  UseLocalSolver=off  LocalSolverChoice=NE_BACKWARD_EULER_ADVANCER  LocalSolverSampleTime=0.001  DoFixedCost=off  MaxNonlinIter=3  MaxModeIter=2  ComputeImpulses=off  ImpulseIterations=2  LinearAlgebra=Sparse  EquationFormulation=NE_TIME_EF  DelaysMemoryBudget=1024  AutomaticFiltering=on  FilteringTimeConstant=0.001  PartitionStorageMethod=AS_NEEDED  PartitionMemoryBudget=1024  PartitionMethod=FAST
      settings: SourceProductBaseCode=PW,SS
  World Frame : sm_lib/Frames and Transforms/World Frame
  Origin : PMIOPort  Side=Right
  connections:
  Solver Configuration/RConn1 -- World Frame/RConn1 -- Mechanism Configuration1/RConn1 -- Origin/RConn1

== system GreenCraneSimulator_SomplifiedHydMechModel/PC | Ubuntu | ROS2/Green Crane | Visualizer  ==
  thetaBoom : Inport
  Boom : sm_lib/Body Elements/File Solid  ExtGeomFileName=..\MAS418_SimulinkModel\CAD\Boom.STL  UnitType=Custom  ExtGeomFileUnits=mm  StepReaderType=HEX  ExportConvexHullGeometry=off  InertiaType=CalculateFromGeometry  Mass=1  MassUnits=kg  CenterOfMass=[0 0 0]  CenterOfMassUnits=m  MomentsOfInertia=[1 1 1]  MomentsOfInertiaUnits=kg*m^2  ProductsOfInertia=[0 0 0]  ProductsOfInertiaUnits=kg*m^2  BasedOnType=Density  Density=1000  DensityUnits=kg/m^3  DoExposeReferenceFrame=off  SerializedFrames=<Frames><Frame><Id>Frame1</Id><Value><Name>F1</Name><Origin><Source>CenterOfMassFrame</Source><FeatureName></FeatureName></Origin><PrimaryAxis><DefinedDirection>+Y</DefinedDirection><Source>ReferenceFrame</Source><SourceDirection>-Z</SourceDirection><FeatureName></FeatureName></PrimaryAxis><SecondaryAxis><DefinedDirection>+X</DefinedDirection><Source>ReferenceFrame</Source><SourceDirection>+X</SourceDirection><FeatureName></FeatureName></SecondaryAxis></Value></Frame></Frames>  GraphicType=FromGeometry  MarkerShape=Sphere  MarkerSize=10  GraphicVisPropType=SimpleVisualProperties  GraphicDiffuseColor=[0.0 0.4 0.0]  GraphicSpecularColor=[0.5 0.5 0.5 1.0]  GraphicAmbientColor=[0.15 0.15 0.15 1.0]  GraphicEmissiveColor=[0.0 0.0 0.0 1.0]  GraphicShininess=75  GraphicOpacity=1.0
  Frame : sm_lib/Body Elements/File Solid  ExtGeomFileName=..\MAS418_SimulinkModel\CAD\Frame.STL  UnitType=Custom  ExtGeomFileUnits=mm  StepReaderType=HEX  ExportConvexHullGeometry=off  InertiaType=CalculateFromGeometry  Mass=1  MassUnits=kg  CenterOfMass=[0 0 0]  CenterOfMassUnits=m  MomentsOfInertia=[1 1 1]  MomentsOfInertiaUnits=kg*m^2  ProductsOfInertia=[0 0 0]  ProductsOfInertiaUnits=kg*m^2  BasedOnType=Density  Density=1000  DensityUnits=kg/m^3  DoExposeReferenceFrame=off  SerializedFrames=<Frames><Frame><Id>Frame1</Id><Value><Name>F1</Name><Origin><Source>CenterOfMassFrame</Source><FeatureName></FeatureName></Origin><PrimaryAxis><DefinedDirection>-Y</DefinedDirection><Source>ReferenceFrame</Source><SourceDirection>+Z</SourceDirection><FeatureName></FeatureName></PrimaryAxis><SecondaryAxis><DefinedDirection>+X</DefinedDirection><Source>ReferenceFrame</Source><SourceDirection>+X</SourceDirection><FeatureName></FeatureName></SecondaryAxis></Value></Frame></Frames>  GraphicType=FromGeometry  MarkerShape=Sphere  MarkerSize=10  GraphicVisPropType=SimpleVisualProperties  GraphicDiffuseColor=[0.0 0.4 0.0]  GraphicSpecularColor=[0.5 0.5 0.5 1.0]  GraphicAmbientColor=[0.15 0.15 0.15 1.0]  GraphicEmissiveColor=[0.0 0.0 0.0 1.0]  GraphicShininess=75  GraphicOpacity=1.0
  RJ Boom : sm_lib/Joints/Revolute Joint  JointMode=Normal  SenseConstraintForce=off  SenseConstraintForceX=off  SenseConstraintForceY=off  SenseConstraintForceZ=off  SenseConstraintTorque=off  SenseConstraintTorqueX=off  SenseConstraintTorqueY=off  SenseConstraintTorqueZ=off  SenseTotalForce=off  SenseTotalForceX=off  SenseTotalForceY=off  SenseTotalForceZ=off  SenseTotalTorque=off  SenseTotalTorqueX=off  SenseTotalTorqueY=off  SenseTotalTorqueZ=off  CompositeWrenchDir=FollowerOnBase  CompositeWrenchFrame=BaseFrame  EquilibriumPosition=0  EquilibriumPositionUnits=deg  SpringStiffness=0  SpringStiffnessUnits=N*m/deg  DampingCoefficient=0  DampingCoefficientUnits=N*m/(deg/s)  TorqueActuationMode=ComputedTorque  MotionActuationMode=InputMotion  SensePosition=off  SenseVelocity=off  SenseAcceleration=off  SenseTorqueForce=off  SenseLowerLimitTorqueForce=off  SenseUpperLimitTorqueForce=off  LowerLimitSpecify=off  LowerLimitBound=-90  LowerLimitBoundUnits=deg  LowerLimitStiffness=1e4  LowerLimitStiffnessUnits=N*m/deg  LowerLimitDamping=10  LowerLimitDampingUnits=N*m/(deg/s)  LowerLimitTransitionRegionWidth=0.1  LowerLimitTransitionRegionWidthUnits=deg  UpperLimitSpecify=off  UpperLimitBound=90  UpperLimitBoundUnits=deg  UpperLimitStiffness=1e4  UpperLimitStiffnessUnits=N*m/deg  UpperLimitDamping=10  UpperLimitDampingUnits=N*m/(deg/s)  UpperLimitTransitionRegionWidth=0.1  UpperLimitTransitionRegionWidthUnits=deg  PositionTargetSpecify=off  PositionTargetPriority=High  PositionTargetValue=0.326727675  PositionTargetValueUnits=rad  VelocityTargetSpecify=off  VelocityTargetPriority=High  VelocityTargetValue=0  VelocityTargetValueUnits=deg/s
  Rigid Transform : sm_lib/Frames and Transforms/Rigid Transform  TranslationMethod=Cartesian  TranslationStandardOffset=0  TranslationLengthUnit=mm  TranslationStandardAxis=+Z  TranslationCartesianOffset=[-568.76 0 1179.93]  TranslationROffset=0  TranslationROffsetUnits=m  TranslationZOffset=0  TranslationZOffsetUnits=m  TranslationThetaOffset=0  TranslationThetaOffsetUnits=deg  RotationMethod=StandardAxis  RotationAngleUnits=deg  RotationStandardAxis=+X  RotationAngle=90  RotationArbitraryAxis=[0 0 1]  FollAlignAxisA=+X  BaseAlignAxisA=+Y  FollAlignAxisB=+Y  BaseAlignAxisB=+Z  RotationSequenceAxes=FollowerAxes  RotationSequence=XYX  RotationSequenceAngles=[0 0 0]  RotationSequenceAnglesUnits=deg  RotationMatrix=[1 0 0; 0 1 0; 0 0 1]
  Rigid Transform1 : sm_lib/Frames and Transforms/Rigid Transform  TranslationMethod=Cartesian  TranslationStandardOffset=0  TranslationLengthUnit=mm  TranslationStandardAxis=+Z  TranslationCartesianOffset=[-3108.36 0 -63.43]  TranslationROffset=0  TranslationROffsetUnits=m  TranslationZOffset=0  TranslationZOffsetUnits=m  TranslationThetaOffset=0  TranslationThetaOffsetUnits=deg  RotationMethod=StandardAxis  RotationAngleUnits=deg  RotationStandardAxis=+X  RotationAngle=90  RotationArbitraryAxis=[0 0 1]  FollAlignAxisA=+X  BaseAlignAxisA=+Y  FollAlignAxisB=+Y  BaseAlignAxisB=+Z  RotationSequenceAxes=FollowerAxes  RotationSequence=XYX  RotationSequenceAngles=[0 0 0]  RotationSequenceAnglesUnits=deg  RotationMatrix=[1 0 0; 0 1 0; 0 0 1]
  Setup : Subsystem
  Simulink-PS Converter : nesl_utility/Simulink-PS Converter  PhysicalDomain=network_engine_domain  SubClassName=ps_input  LeftPortType=input  RightPortType=output  PseudoPeriodic=off  Frequencies=[]  NoiseDistribution=none  NoiseParameters=[]  Unit=1  AffineConversion=off  FilteringAndDerivatives=filter  SimscapeFilterOrder=2  InputFilterTimeConstant=0.001  UdotUserProvided=0
      settings: SourceProductBaseCode=PW,SS
  wires:
  thetaBoom/1 -> Simulink-PS Converter/1
  connections:
  Setup/RConn1 -- Rigid Transform/LConn1 -- Frame/LConn1
  Rigid Transform1/LConn1 -- Boom/LConn1
  RJ Boom/LConn1 -- Rigid Transform/RConn1
  RJ Boom/RConn1 -- Rigid Transform1/RConn1
  Simulink-PS Converter/RConn1 -- RJ Boom/LConn2

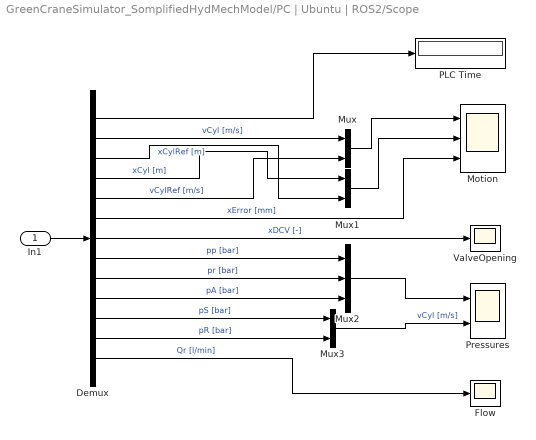
== system GreenCraneSimulator_SomplifiedHydMechModel/PC | Ubuntu | ROS2/Scope ==
  In1 : Inport
  Demux : Demux  Outputs=13
  Flow : Scope
  Motion : Scope  NumInputPorts=3
  Mux : Mux  Inputs=2
  Mux1 : Mux  Inputs=2
  Mux2 : Mux  Inputs=3
  Mux3 : Mux  Inputs=2
  PLC Time : Display
  Pressures : Scope  NumInputPorts=2
  ValveOpening : Scope
  wires:
  Demux/4 -> Mux1/1  "xCyl [m]"
  Mux/1 -> Motion/1
  Demux/5 -> Mux/2  "vCylRef [m/s]"
  Demux/9 -> Mux2/2  "pr [bar]"
  Demux/3 -> Mux1/2  "xCylRef [m]"
  Mux1/1 -> Motion/2
  Demux/8 -> Mux2/1  "pp [bar]"
  Demux/7 -> ValveOpening/1  "xDCV [-]"
  Demux/2 -> Mux/1  "vCyl [m/s]"
  Demux/6 -> Motion/3  "xError [mm]"
  In1/1 -> Demux/1
  Demux/1 -> PLC Time/1
  Demux/10 -> Mux2/3  "pA [bar]"
  Mux2/1 -> Pressures/1
  Mux3/1 -> Pressures/2  "vCyl [m/s]"
  Demux/11 -> Mux3/1  "pS [bar]"
  Demux/12 -> Mux3/2  "pR [bar]"
  Demux/13 -> Flow/1  "Qr [l/min]"

== system GreenCraneSimulator_SomplifiedHydMechModel/PLC/Discrete Derivative ==
  xCyl [m] : Inport
  Discrete Derivative : simulink/Discrete/Discrete Derivative  gainval=1.0  ICPrevScaledInput=0  OutMin=[]  OutMax=[]  OutDataType=fixdt(1, 16)  OutScaling=2^-10  DoSatur=off
  Saturation : Saturate
  Zero-Order Hold : ZeroOrderHold  SampleTime=-1
  vCyl [m/s] : Outport
  wires:
  Discrete Derivative/1 -> Saturation/1  "vCyl [m/s]"
  Zero-Order Hold/1 -> Discrete Derivative/1
  xCyl [m]/1 -> Zero-Order Hold/1
  Saturation/1 -> vCyl [m/s]/1  "vCyl [m/s]"

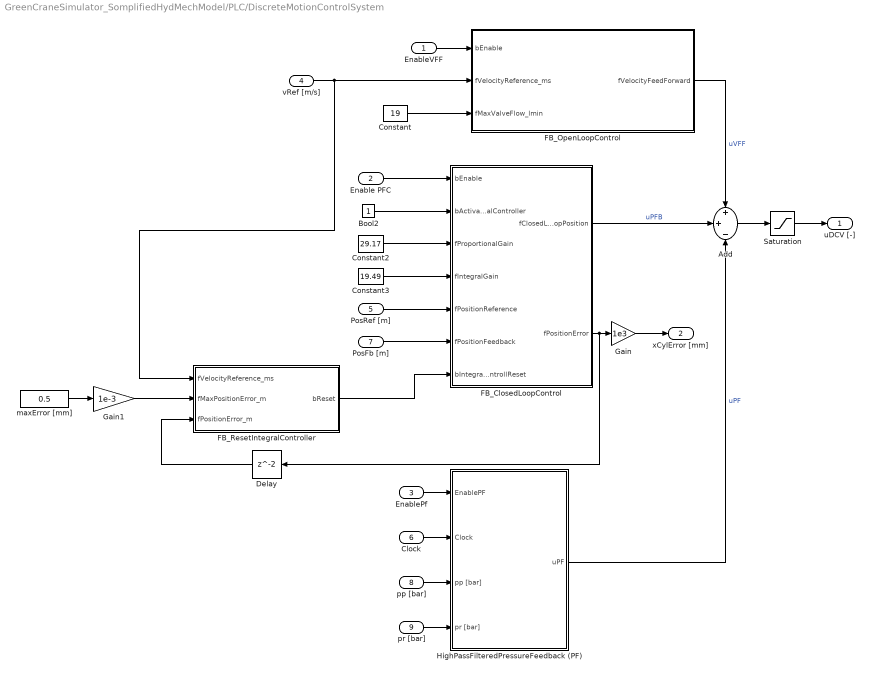
== system GreenCraneSimulator_SomplifiedHydMechModel/PLC/DiscreteMotionControlSystem ==
  EnableVFF : Inport
  Enable PFC : Inport  Port=2
  EnablePf : Inport  Port=3
  vRef [m/s] : Inport  Port=4
  PosRef [m] : Inport  Port=5
  Clock : Inport  Port=6
  PosFb [m] : Inport  Port=7
  pp [bar] : Inport  Port=8
  pr [bar] : Inport  Port=9
  Add : Sum  Inputs=++-
  Bool2 : Constant  OutDataTypeStr=boolean
  Constant : Constant  Value=19
  Constant2 : Constant  Value=29.17
  Constant3 : Constant  Value=19.49
  Delay : Delay
  FB_ClosedLoopControl : Subsystem  TreatAsAtomicUnit=on
  FB_OpenLoopControl : Subsystem  TreatAsAtomicUnit=on
  FB_ResetIntegralController : Subsystem  TreatAsAtomicUnit=on
  Gain : Gain  Gain=1e3
  Gain1 : Gain  Gain=1e-3
  HighPassFilteredPressureFeedback (PF) : Subsystem  TreatAsAtomicUnit=on  SystemSampleTime=tCycle
  Saturation : Saturate  UpperLimit=1  LowerLimit=-1
  maxError [mm] : Constant  Value=0.5
  uDCV [-] : Outport
  xCylError [mm] : Outport  Port=2
  wires:
  Constant2/1 -> FB_ClosedLoopControl/3(fProportionalGain)
  Enable PFC/1 -> FB_ClosedLoopControl/1(bEnable)
  Constant3/1 -> FB_ClosedLoopControl/4(fIntegralGain)
  EnableVFF/1 -> FB_OpenLoopControl/1(bEnable)
  Bool2/1 -> FB_ClosedLoopControl/2(bActivateIntegralController)
  FB_ClosedLoopControl/2(fPositionError) -> Delay/1, Gain/1
  HighPassFilteredPressureFeedback (PF)/1(uPF) -> Add/3  "uPF"
  Constant/1 -> FB_OpenLoopControl/3(fMaxValveFlow_lmin)
  FB_OpenLoopControl/1(fVelocityFeedForward) -> Add/1  "uVFF"
  FB_ClosedLoopControl/1(fClosedLoopPosition) -> Add/2  "uPFB"
  PosFb [m]/1 -> FB_ClosedLoopControl/6(fPositionFeedback)
  PosRef [m]/1 -> FB_ClosedLoopControl/5(fPositionReference)
  EnablePf/1 -> HighPassFilteredPressureFeedback (PF)/1(EnablePF)
  Clock/1 -> HighPassFilteredPressureFeedback (PF)/2(Clock)
  pp [bar]/1 -> HighPassFilteredPressureFeedback (PF)/3(pp [bar])
  pr [bar]/1 -> HighPassFilteredPressureFeedback (PF)/4(pr [bar])
  Add/1 -> Saturation/1
  Gain/1 -> xCylError [mm]/1
  maxError [mm]/1 -> Gain1/1
  Saturation/1 -> uDCV [-]/1
  FB_ResetIntegralController/1(bReset) -> FB_ClosedLoopControl/7(bIntegralControllReset)
  Delay/1 -> FB_ResetIntegralController/3(fPositionError_m)
  Gain1/1 -> FB_ResetIntegralController/2(fMaxPositionError_m)
  vRef [m/s]/1 -> FB_OpenLoopControl/2(fVelocityReference_ms), FB_ResetIntegralController/1(fVelocityReference_ms)

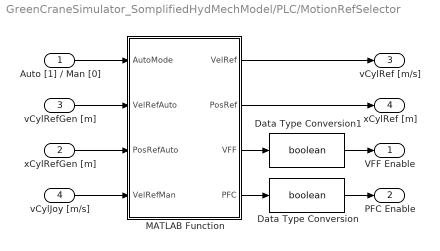
== system GreenCraneSimulator_SomplifiedHydMechModel/PLC/MotionRefSelector ==
  Auto [1] / Man [0] : Inport  OutDataTypeStr=boolean
  xCylRefGen [m] : Inport  Port=2
  vCylRefGen [m] : Inport  Port=3
  vCylJoy [m/s] : Inport  Port=4
  Data Type Conversion : DataTypeConversion  OutDataTypeStr=boolean
  Data Type Conversion1 : DataTypeConversion  OutDataTypeStr=boolean
  MATLAB Function : MATLAB Function  TreatAsAtomicUnit=on
  VFF Enable : Outport  OutDataTypeStr=boolean
  PFC Enable : Outport  Port=2  OutDataTypeStr=boolean
  vCylRef [m/s] : Outport  Port=3
  xCylRef [m] : Outport  Port=4
  wires:
  Auto [1] / Man [0]/1 -> MATLAB Function/1(AutoMode)
  vCylJoy [m/s]/1 -> MATLAB Function/4(VelRefMan)
  xCylRefGen [m]/1 -> MATLAB Function/3(PosRefAuto)
  vCylRefGen [m]/1 -> MATLAB Function/2(VelRefAuto)
  MATLAB Function/1(VelRef) -> vCylRef [m/s]/1
  MATLAB Function/2(PosRef) -> xCylRef [m]/1
  MATLAB Function/3(VFF) -> Data Type Conversion1/1
  MATLAB Function/4(PFC) -> Data Type Conversion/1
  Data Type Conversion/1 -> PFC Enable/1
  Data Type Conversion1/1 -> VFF Enable/1

== system GreenCraneSimulator_SomplifiedHydMechModel/PLC/MotionReferenceTime ==
  <StartAuto> : Inport
  <StopAuto> : Inport  Port=2
  Constant : Constant
  Discrete-Time Integrator : DiscreteIntegrator  SampleTime=-1  ICPrevOutput=DiscIntNeverNeededParam  ICPrevScaledInput=DiscIntNeverNeededParam
  MATLAB Function : MATLAB Function  TreatAsAtomicUnit=on
  Time : Outport
  wires:
  <StartAuto>/1 -> MATLAB Function/1(StartClock)
  <StopAuto>/1 -> MATLAB Function/2(StopClock)
  Constant/1 -> Discrete-Time Integrator/1
  MATLAB Function/1(Time) -> Time/1
  Discrete-Time Integrator/1 -> MATLAB Function/3(Clock)

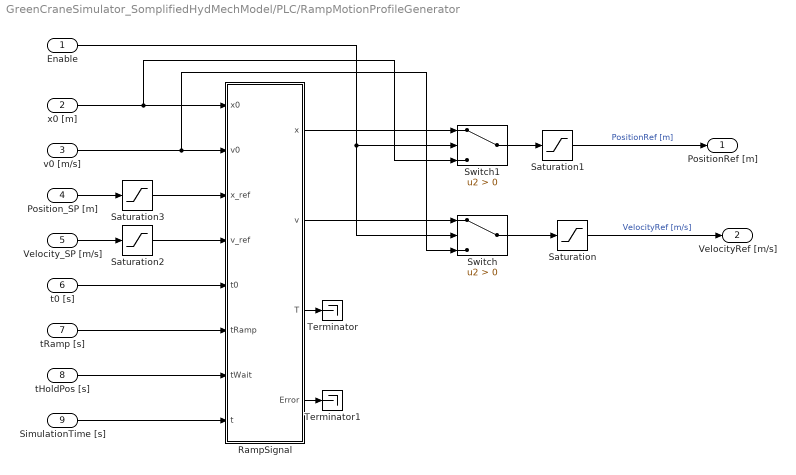
== system GreenCraneSimulator_SomplifiedHydMechModel/PLC/RampMotionProfileGenerator ==
  Enable : Inport  OutDataTypeStr=boolean
  x0 [m] : Inport  Port=2  OutDataTypeStr=double
  v0 [m/s] : Inport  Port=3  OutDataTypeStr=double
  Position_SP [m] : Inport  Port=4  OutDataTypeStr=double
  "Velocity_SP [m/s] " : Inport  Port=5  OutDataTypeStr=double
  t0 [s] : Inport  Port=6  OutDataTypeStr=double
  tRamp [s] : Inport  Port=7  OutDataTypeStr=double
  tHoldPos [s] : Inport  Port=8  OutDataTypeStr=double
  SimulationTime [s] : Inport  Port=9  OutDataTypeStr=double
  RampSignal : MATLAB Function  TreatAsAtomicUnit=on
  Saturation : Saturate  UpperLimit=150  LowerLimit=-150
  Saturation1 : Saturate  UpperLimit=500  LowerLimit=0
  Saturation2 : Saturate  UpperLimit=0.120  LowerLimit=0
  Saturation3 : Saturate  LowerLimit=0
  Switch : Switch  Criteria=u2 > Threshold
  Switch1 : Switch  Criteria=u2 > Threshold
  Terminator : Terminator
  Terminator1 : Terminator
  "PositionRef [m] " : Outport  VectorParamsAs1DForOutWhenUnconnected=off
  VelocityRef [m/s] : Outport  Port=2  VectorParamsAs1DForOutWhenUnconnected=off
  wires:
  SimulationTime [s]/1 -> RampSignal/8(t)
  RampSignal/2(v) -> Switch/1
  Switch/1 -> Saturation/1
  v0 [m/s]/1 -> RampSignal/2(v0), Switch/3
  t0 [s]/1 -> RampSignal/5(t0)
  Position_SP [m]/1 -> Saturation3/1
  tHoldPos [s]/1 -> RampSignal/7(tWait)
  "Velocity_SP [m/s] "/1 -> Saturation2/1
  RampSignal/1(x) -> Switch1/1
  Enable/1 -> Switch/2, Switch1/2
  x0 [m]/1 -> Switch1/3, RampSignal/1(x0)
  Switch1/1 -> Saturation1/1
  Saturation2/1 -> RampSignal/4(v_ref)
  Saturation3/1 -> RampSignal/3(x_ref)
  tRamp [s]/1 -> RampSignal/6(tRamp)
  RampSignal/3(T) -> Terminator/1
  RampSignal/4(Error) -> Terminator1/1
  Saturation1/1 -> "PositionRef [m] "/1  "PositionRef [m]"
  Saturation/1 -> VelocityRef [m/s]/1  "VelocityRef [m/s]"

== system GreenCraneSimulator_SomplifiedHydMechModel/PC | Ubuntu | ROS2/Green Crane | Visualizer /Setup ==
  Mechanism Configuration1 : sm_lib/Utilities/Mechanism Configuration  UniformGravity=Constant  GravityVector=[0 0 -9.80665]  GravityUnits=m/s^2  LinearizationDelta=0.001  JointModeTransitionNonlinearIterations=2
  Solver Configuration : nesl_utility/Solver Configuration  PhysicalDomain=network_engine_domain  SubClassName=solver  LeftPortType=input  RightPortType=generic  Tones=[]  Harmonics=[]  SimulateNoise=off  Profile=off  UseLocalSampling=off  EnableSwitchedLinearOptims=on  FrequencyDomain=off  UseCCode=off  RelTol=0.001  AbsTol=1e-06  MinStep=1e-09  ToWorkspace=off  RevertToSquareIcSolve=off  NumHomotopyIterations=100  PhasorMode=off  PhasorModeNumHarmonics=1  DoDC=off  ResidualTolerance=1e-09  UseLocalSolver=off  LocalSolverChoice=NE_BACKWARD_EULER_ADVANCER  LocalSolverSampleTime=0.001  DoFixedCost=off  MaxNonlinIter=3  MaxModeIter=2  ComputeImpulses=off  ImpulseIterations=2  LinearAlgebra=Sparse  EquationFormulation=NE_TIME_EF  DelaysMemoryBudget=1024  AutomaticFiltering=on  FilteringTimeConstant=0.001  PartitionStorageMethod=AS_NEEDED  PartitionMemoryBudget=1024  PartitionMethod=FAST
      settings: SourceProductBaseCode=PW,SS
  World Frame : sm_lib/Frames and Transforms/World Frame
  Origin : PMIOPort  Side=Right
  connections:
  Solver Configuration/RConn1 -- World Frame/RConn1 -- Mechanism Configuration1/RConn1 -- Origin/RConn1

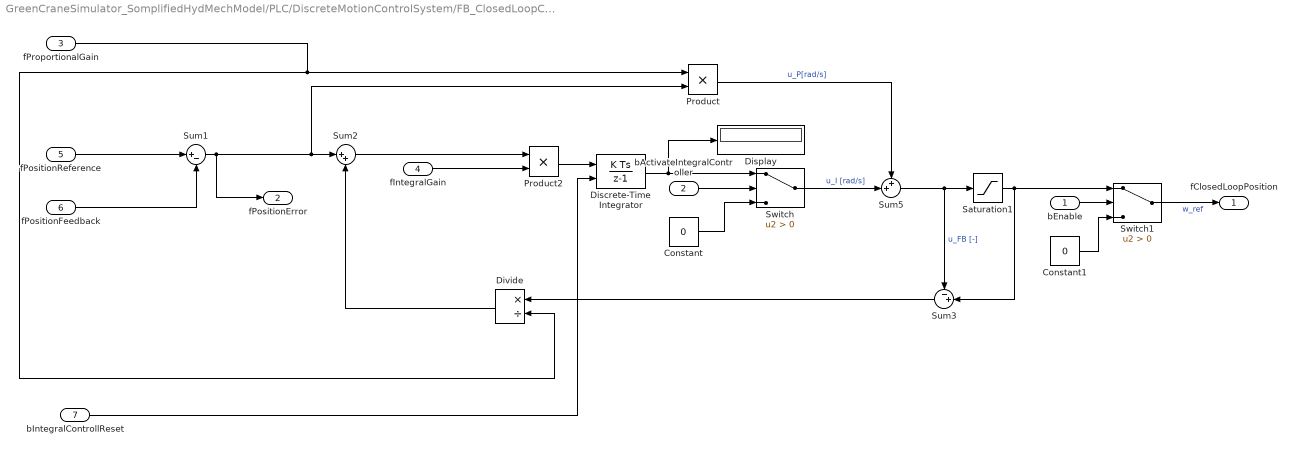
== system GreenCraneSimulator_SomplifiedHydMechModel/PLC/DiscreteMotionControlSystem/FB_ClosedLoopControl ==
  bEnable : Inport  OutDataTypeStr=boolean
  bActivateIntegralController : Inport  Port=2  OutDataTypeStr=boolean
  fProportionalGain : Inport  Port=3
  fIntegralGain : Inport  Port=4
  fPositionReference : Inport  Port=5
  fPositionFeedback : Inport  Port=6
  bIntegralControllReset : Inport  Port=7  OutDataTypeStr=boolean
  Constant : Constant  Value=0
  Constant1 : Constant  Value=0
  Discrete-Time Integrator : DiscreteIntegrator  ExternalReset=sampled level  SampleTime=-1  LimitOutput=on  UpperSaturationLimit=1  LowerSaturationLimit=-1  ICPrevOutput=DiscIntNeverNeededParam  ICPrevScaledInput=DiscIntNeverNeededParam
  Display : Display
  Divide : Product  Inputs=*/
  Product : Product
  Product2 : Product
  Saturation1 : Saturate  UpperLimit=1  LowerLimit=-1
  Sum1 : Sum  Inputs=|+-
  Sum2 : Sum  Inputs=|++
  Sum3 : Sum  Inputs=-+|
  Sum5 : Sum  Inputs=++|
  Switch : Switch  Criteria=u2 > Threshold
  Switch1 : Switch  Criteria=u2 > Threshold
  fClosedLoopPosition : Outport  VectorParamsAs1DForOutWhenUnconnected=off
  fPositionError : Outport  Port=2  VectorParamsAs1DForOutWhenUnconnected=off
  wires:
  fPositionFeedback/1 -> Sum1/2
  Sum2/1 -> Product2/1
  Divide/1 -> Sum2/2
  fProportionalGain/1 -> Product/1, Divide/2
  fIntegralGain/1 -> Product2/2
  bActivateIntegralController/1 -> Switch/2
  Constant/1 -> Switch/3
  fPositionReference/1 -> Sum1/1
  Sum5/1 -> Sum3/1, Saturation1/1  "u_FB [-]"
  Sum3/1 -> Divide/1
  Switch1/1 -> fClosedLoopPosition/1  "w_ref"
  Constant1/1 -> Switch1/3
  bEnable/1 -> Switch1/2
  Saturation1/1 -> Switch1/1, Sum3/2
  Product/1 -> Sum5/1  "u_P[rad/s]"
  Switch/1 -> Sum5/2  "u_I [rad/s]"
  Product2/1 -> Discrete-Time Integrator/1
  bIntegralControllReset/1 -> Discrete-Time Integrator/2
  Discrete-Time Integrator/1 -> Display/1, Switch/1
  Sum1/1 -> fPositionError/1, Product/2, Sum2/1

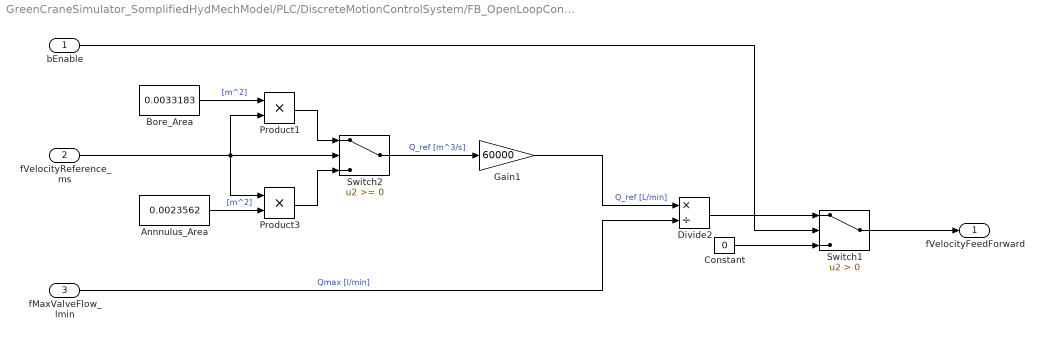
== system GreenCraneSimulator_SomplifiedHydMechModel/PLC/DiscreteMotionControlSystem/FB_OpenLoopControl ==
  bEnable : Inport  OutDataTypeStr=boolean
  fVelocityReference_ms : Inport  Port=2
  fMaxValveFlow_lmin : Inport  Port=3
  Annnulus_Area : Constant  Value=0.0023562
  Bore_Area : Constant  Value=0.0033183
  Constant : Constant  Value=0
  Divide2 : Product  Inputs=*/
  Gain1 : Gain  Gain=60000
  Product1 : Product
  Product3 : Product
  Switch1 : Switch  Criteria=u2 > Threshold
  Switch2 : Switch
  fVelocityFeedForward : Outport  VectorParamsAs1DForOutWhenUnconnected=off
  wires:
  Annnulus_Area/1 -> Product3/2  "[m^2]"
  Switch2/1 -> Gain1/1  "Q_ref [m^3/s]"
  Product1/1 -> Switch2/1
  fVelocityReference_ms/1 -> Product3/1, Product1/2, Switch2/2
  fMaxValveFlow_lmin/1 -> Divide2/2  "Qmax [l/min]"
  Bore_Area/1 -> Product1/1  "[m^2]"
  Gain1/1 -> Divide2/1  "Q_ref [L/min]"
  Product3/1 -> Switch2/3
  Constant/1 -> Switch1/3
  Divide2/1 -> Switch1/1
  bEnable/1 -> Switch1/2
  Switch1/1 -> fVelocityFeedForward/1

== system GreenCraneSimulator_SomplifiedHydMechModel/PLC/DiscreteMotionControlSystem/FB_ResetIntegralController ==
  fVelocityReference_ms : Inport
  fMaxPositionError_m : Inport  Port=2
  fPositionError_m : Inport  Port=3
  Data Type Conversion : DataTypeConversion  OutDataTypeStr=boolean
  ResetIntegralController : MATLAB Function  TreatAsAtomicUnit=on
  bReset : Outport  OutDataTypeStr=boolean
  wires:
  fMaxPositionError_m/1 -> ResetIntegralController/2(exCylMax)
  fVelocityReference_ms/1 -> ResetIntegralController/1(vRef)
  ResetIntegralController/1(Reset) -> Data Type Conversion/1
  fPositionError_m/1 -> ResetIntegralController/3(exCyl)
  Data Type Conversion/1 -> bReset/1
